simulink model "retour_etat_integral"  (R2023b)
settings: Solver=VariableStepAuto  StartTime=0.0  StopTime=70  MaxStep=1e-4  RelTol=1e-3
values from neighbouring files (symbols this model uses):
  delta0 = n_g / K_s * Tg0    [EI.m]
  K_I = K(:,4)    [EI.m]
  K_x = K(:,1:3)    [EI.m]
undefined symbols (not defined in the file or in its folder): x
settings Model: Creator=33783  LastModifiedBy=33783

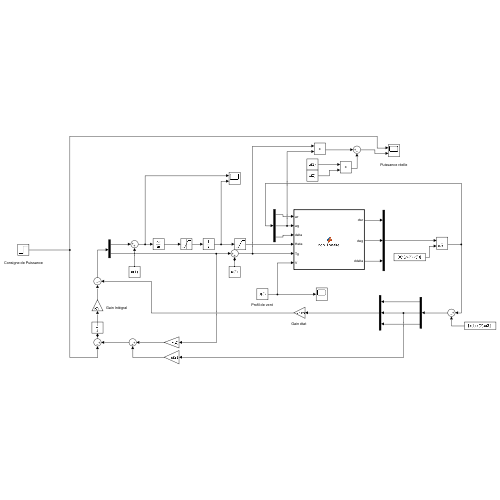
[thumbnail: Simulink's stored preview of the top-level diagram]
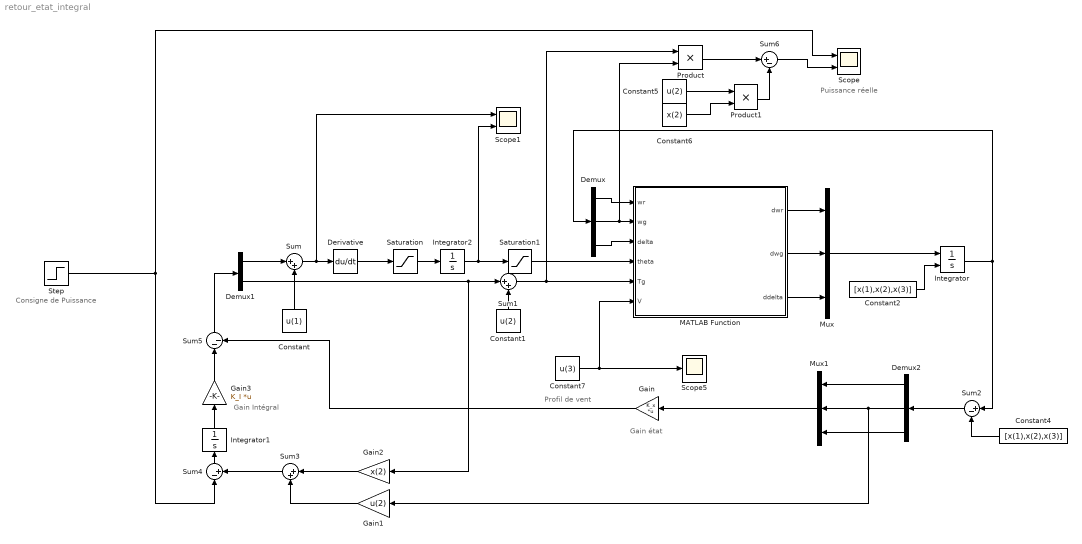
== system retour_etat_integral ==
  note: Puissance réelle
  note: Profil de vent
  note: Gain état
  note: Gain Intégral
  note: Consigne de Puissance
  Constant : Constant  Value=u(1)
  Constant1 : Constant  Value=u(2)
  Constant2 : Constant  Value=[x(1),x(2),x(3)]  VectorParams1D=off
  Constant4 : Constant  Value=[x(1),x(2),x(3)]  VectorParams1D=off
  Constant5 : Constant  Value=u(2)
  Constant6 : Constant  Value=x(2)
  Constant7 : Constant  Value=u(3)
  Demux : Demux  Outputs=3
  Demux1 : Demux  Outputs=2
  Demux2 : Demux  Outputs=3
  Derivative : Derivative
  Gain : Gain  Gain=K_x  Multiplication=Matrix(K*u) (u vector)
  Gain1 : Gain  Gain=u(2)
  Gain2 : Gain  Gain=x(2)
  Gain3 : Gain  Gain=K_I  Multiplication=Matrix(K*u)
  Integrator : Integrator  InitialConditionSource=external  InitialCondition=[4.267,184.2,delta0]
  Integrator1 : Integrator
  Integrator2 : Integrator  InitialCondition=u(1)
  MATLAB Function : MATLAB Function  TreatAsAtomicUnit=on
  Mux : Mux  Inputs=3
  Mux1 : Mux  Inputs=3
  Product : Product
  Product1 : Product
  Saturation : Saturate  UpperLimit=19  LowerLimit=-19
  Saturation1 : Saturate  UpperLimit=30  LowerLimit=-5
  Scope : Scope  NumInputPorts=2
  Scope1 : Scope  NumInputPorts=2
  Scope5 : Scope
  Step : Step  Time=5  After=+10000  SampleTime=0
  Sum : Sum  Inputs=|++
  Sum1 : Sum  Inputs=|++
  Sum2 : Sum  Inputs=|+-
  Sum3 : Sum  Inputs=|++
  Sum4 : Sum  Inputs=|-+
  Sum5 : Sum  Inputs=|--
  Sum6 : Sum  Inputs=|+-
  wires:
  MATLAB Function/1(dwr) -> Mux/1
  MATLAB Function/2(dwg) -> Mux/2
  Demux/1 -> MATLAB Function/1(wr)
  Demux/2 -> Product/2, MATLAB Function/2(wg)
  Demux/3 -> MATLAB Function/3(delta)
  MATLAB Function/3(ddelta) -> Mux/3
  Mux/1 -> Integrator/1
  Constant2/1 -> Integrator/2
  Integrator/1 -> Sum2/1, Demux/1
  Sum/1 -> Scope1/1, Derivative/1
  Sum1/1 -> Product/1, MATLAB Function/5(Tg)
  Constant/1 -> Sum/2
  Constant1/1 -> Sum1/2
  Constant4/1 -> Sum2/2
  Gain/1 -> Sum5/2
  Sum2/1 -> Demux2/1
  Demux2/2 -> Gain1/1, Mux1/2
  Demux2/3 -> Mux1/3
  Mux1/1 -> Gain/1
  Gain2/1 -> Sum3/1
  Gain1/1 -> Sum3/2
  Sum3/1 -> Sum4/2
  Sum4/1 -> Integrator1/1
  Integrator1/1 -> Gain3/1
  Gain3/1 -> Sum5/1
  Demux1/1 -> Sum/1
  Demux1/2 -> Gain2/1, Sum1/1
  Sum5/1 -> Demux1/1
  Product/1 -> Sum6/1
  Sum6/1 -> Scope/2
  Product1/1 -> Sum6/2
  Constant5/1 -> Product1/1
  Constant6/1 -> Product1/2
  Step/1 -> Sum4/1, Scope/1
  Saturation/1 -> Integrator2/1
  Derivative/1 -> Saturation/1
  Integrator2/1 -> Saturation1/1, Scope1/2
  Demux2/1 -> Mux1/1
  Saturation1/1 -> MATLAB Function/4(theta)
  Constant7/1 -> MATLAB Function/6(V), Scope5/1

== matlab function retour_etat_integral/MATLAB Function ==
  data: wr input; dwr output; wg input; delta input; theta input; Tg input; dwg output; ddelta output; V input
function [dwr,dwg,ddelta] = non_lineaire(wr,wg,delta,theta,Tg,V)
    % Valeurs du modèle :
    n_g = 43.165 ; % sans unité
    J_r = 3.25e5; % kg/m^2
    J_g = 34.4 ; % kg/m^2
    K_s = 269.1e3 ; % N.m/rad
    R = 21.65 ; % en mètres
    rho = 1.225 ; % en kg/m3
    D_s= 9500; % Nm/rad/s
    
    function Lambdai = funLambdai(lambda,theta)
        Lambdai = 1/(1/(lambda+0.08*theta)- 0.035/(theta^3 + 1)) ;
    end
    
    function Cp = funCp(lambda,theta) 
        Cp = 0.5*(116/funLambdai(lambda,theta)-0.4*theta-5)*exp(-21/funLambdai(lambda,theta)) + 0.0068*lambda ;
    end

    function Pr = funPuissance(wr,theta,V)
        Pr = 0.5*rho*pi*(R^2)*(V^3)*funCp(wr*R/V,theta);
    end
    
    dwr = 1/(J_r*wr) * funPuissance(wr,theta,V) - (D_s/J_r) *  + (wr*D_s/(J_r*n_g)) * wg - (K_s/J_r) * delta ;
    dwg = (D_s/(J_g * n_g)) * wr - (D_s/(J_g * n_g^2)) * wg + (K_s/(J_g * n_g)) * delta - (1/J_g) * Tg ;
    ddelta = wr - 1/n_g * wg;
end
